simulink model "ModosDeslizantesPendulo"  (R2022a)
settings: Solver=VariableStepAuto  StartTime=0.0  StopTime=10.0  RelTol=1e-3
settings Model: Creator=benja  LastModifiedBy=benja

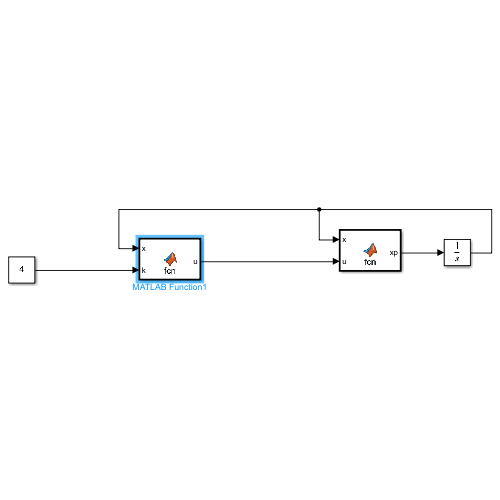
[thumbnail: Simulink's stored preview of the top-level diagram]
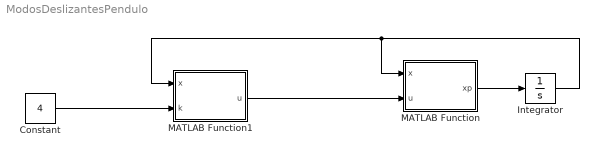
== system ModosDeslizantesPendulo ==
  Constant : Constant  Value=4
  Integrator : Integrator
  MATLAB Function : MATLAB Function  TreatAsAtomicUnit=on
  MATLAB Function1 : MATLAB Function  TreatAsAtomicUnit=on
  wires:
  MATLAB Function/1(xp) -> Integrator/1
  Integrator/1 -> MATLAB Function1/1(x), MATLAB Function/1(x)
  MATLAB Function1/1(u) -> MATLAB Function/2(u)
  Constant/1 -> MATLAB Function1/2(k)

== matlab function ModosDeslizantesPendulo/MATLAB Function ==
  data: x input; u input; xp output
function xp  = fcn(x, u)

a1 = 1
m = 0.1
l = 1
k0 = 0.02
g = 9.81

x1p = x(2)
x2p = -(g/l)*sin(x(1) + d1) - (k0/m)*x(2) + (1/m*l^2)*u

xp = [x1p x2p]

== matlab function ModosDeslizantesPendulo/MATLAB Function1 ==
  data: x input; u output; k input
function u = fcn(x,k)
a1 = 1

u = -k*sign(a*x(1)+x(2))
